simulink library "libBusSerialize"  (R2015a)
settings: Solver=ode45  StartTime=0.0  StopTime=10.0  RelTol=1e-3
undefined symbols (not defined in the file): BusSerialize, macaddr, mxpcnetworkconfig, RigInfo, SimulinkParameter_TestParamPulse, SimulinkParameter_TestParamToggle, SimulinkParameter_TunableConditions, SimulinkParameter_TunableNextTrialId, SimulinkParameter_TunableTaskControl
libraries: simulink x5, xpcethernetlib x3, xpcnetworkbufferlib x2, xpcrtudplib x1
(part 1 of 2)
settings Model: xpc_rtwmakecfg_data=_xpcetherlib__xpcether8255xlib__xpcetherGbElib__xpcnblib__xpciplib_  CovSFcnEnable=off  Creator=shenoylab  LastModifiedBy=shenoylab
settings DebuggingCC: SolverPrmCheckMsg=warning

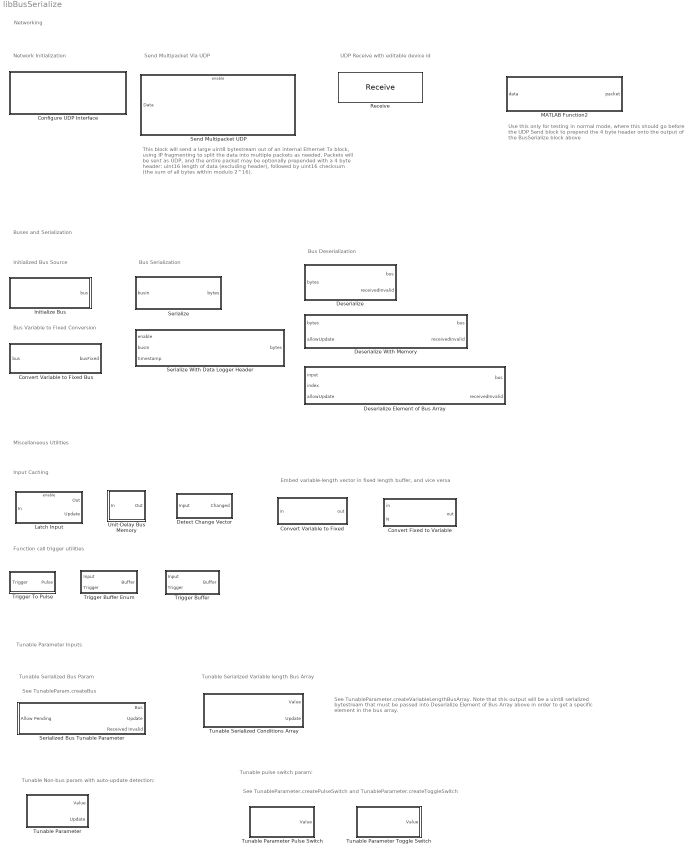
== system libBusSerialize ==
  note: See TunableParameter.createPulseSwitch and TunableParameter.createToggleSwitch
  note: See TunableParam.createBus
  note: See TunableParameter.createVariableLengthBusArray.
      | Note that this output will be a uint8 serialized bytestream that must
      | be passed into Deserialize Element of Bus Array above in order to get a
      | specific element in the bus array.
  note: Use this only for testing in normal mode,
      | where this should go before the UDP Send block
      | to prepend the 4 byte header onto the output of
      | the BusSerialize block above
  note: This block will send a large uint8 bytestream out of an
      | internal Ethernet Tx block, using IP fragmenting to split
      | the data into multiple packets as needed. Packets will be
      | sent as UDP, and the entire packet may be optionally
      | prepended with a 4 byte header: uint16 length of data
      | (excluding header), followed by uint16 checksum (the
      | sum of all bytes within modulo 2^16).
  note: Send Multipacket Via UDP
  note: Bus Serialization
  note: Bus Deserialization
  note: Bus Variable to Fixed Conversion
  note: Input Caching
  note: Function call trigger utilities
  note: Embed variable-length vector in fixed length buffer, and vice versa
  note: Initialized Bus Source
  note: Tunable Non-bus param with auto-update detection:
  note: Tunable pulse switch param:
  note: Tunable Serialized Bus Param
  note: Tunable Serialized Variable length Bus Array
  note: Network Initialization
  note: Networking
  note: Buses and Serialization
  note: Miscellaneous Utilities
  note: Tunable Parameter Inputs
  note: UDP Receive with editable device id
  Configure UDP Interface : Subsystem  InitFcn=mxpcnetworkconfig(1);  mask(xpcnwconfig){PoolSizes=[8196 512 4096 65535], ID=RigInfo.network.hapticVLAN.ethernetId, udpID=0, IpAddress=RigInfo.network.hapticVLAN.sourceIP, SubnetMask=255.255.255.0, Gateway=0.0.0.0, EthDrv=Intel 8255x, PciBus=RigInfo.network.hapticVLAN.pciBus, PciSlot=RigInfo.network.hapticVLAN.pciSlot}
      mask prompts: PoolSizes "Buffer pool sizes (256, 512, 1024, 2048):"; ID "Device ID:"; udpID "Internal UDP ID:"; IpAddress "IP Address:"; SubnetMask "Subnet Mask:"; EthDrv "Ethernet Driver:"; PciBus "PCI Bus:"; PciSlot "PCI Slot:"
      mask help: Configure network interface for real-time UDP communication
      mask init:
      | IpAddress = ipaddr(IpAddress);
      | SubnetMask = ipaddr(SubnetMask);
      | Gateway = ipaddr(Gateway);
      | set_param([gcb '/Ethernet Init '], 'ID', num2str(ID)); % update internal ID, we don't use promotion so the field can be text rather than popup
      | udpID = ID - 1;
      | [MaskDisplay] = mxpcnetworkconfig(2, ID, EthDrv, PciBus, PciSlot);
      | % set_param(gcb, 'MaskDisplay', MaskDisplay);
      mask Help: eval('xpcdoc(''RT_NETWORK_CONFIGURATION'')');
      mask TypeOptions PoolSizes: Buffer Mngmt /PoolSizes
      mask TypeOptions EthDrv: Ethernet Init /Driver
      mask Display:
      | try
      |     ipStr = BusSerialize.ipStringFromAddress(IpAddress);
      |     disp(sprintf('Real-time UDP\nConfiguration\nPCI Bus: %d Slot: %d\nDevice ID: %d\nIP Address: %s', PciBus, PciSlot, ID, ipStr));
      | catch
      |     disp('Real-time UDP\nConfiguration');
      | end
  Convert Fixed to Variable : MATLAB Function  TreatAsAtomicUnit=on  mask(Converts Variable-size to fixed-size array){bufferSize=1500}
      mask prompts: bufferSize "Buffer Size"
      mask help: Specify maximum input size.
  Convert Variable to Fixed : MATLAB Function  TreatAsAtomicUnit=on  mask(Converts Variable-size to fixed-size array){bufferSize=1000}
      mask prompts: bufferSize "Buffer Size"
      mask help: Specify maximum input size.
  Convert Variable to Fixed Bus : MATLAB Function  TreatAsAtomicUnit=on  mask(Drop Variable Length Signals From Bus){busType=Bus: TestBus, busFixedType=Bus: TestBusFixed}
      mask prompts: busType "Bus Type (Input):"; busFixedType "Bus Type (Output):"
      mask help:
      | This block takes as input a bus with some variable length signals, drops all variable length signals from the bus and outputs a bus with the specified type (second drop-down). This is accomplished by calling the appropriate model packaged code function for this bus.
      |
      | See BusSerialize.createBusBaseWorkspaceWithFixedSizeSignalsOnly and BusSerialize.writeDropVariableLengthSignalsFromBusModelPackagedCode.
      mask init:
      | BusSerialize.maskDropVariableLengthSignalsFromBusBlockUpdate(gcb)
  Deserialize : MATLAB Function  TreatAsAtomicUnit=on  mask(BusSerialize: deserialize block){busType=Bus: TestBus}
      mask prompts: busType "Bus Type"
      mask help: Select the bus type below to deserialize into.
      mask init:
      | BusSerialize.maskDeserializeBlockUpdate(gcb)
  Deserialize Element of Bus Array : MATLAB Function  TreatAsAtomicUnit=on  mask(BusSerialize: deserialize a single element of a serialized bus array){busType=Bus: TestBus, inputVariable=off}
      mask prompts: busType "Bus Type:"; inputVariable "Input Variable Length"
      mask help:
      | Given a bus array serialized with BusSerialize.serializeVariableLengthBusArray, this block deserializes a specific element of that bus array. This allows bus arrays to be deserialized even when the bus contains variable length elements (or the array is of variable length), which implies that Simulink cannot currently handle the bus array.
      |
      | Select the bus type below to deserialize into.
      mask init:
      | BusSerialize.maskDeserializeVariableLengthBusArrayBlockUpdate(gcb)
  Deserialize With Memory : MATLAB Function  TreatAsAtomicUnit=on  mask(Deserialize Bus With Internal Memory){busType=Bus: TestBus}
      mask prompts: busType "Bus Type:"
      mask help:
      | This block deserializes a uint8 bytestream into a specific bus type. When the input changes, the block will deserialize the new input, and the deserialization is successful, it will internally store the updated bus.
      |
      | If allowUpdate is high at that point, the new bus value will be output immediately and update will be driven high. If not, pendingUpdate will be driven high, and the updated bus will be held in an internal persistent variable. When allowUpdate goes high, this updated bus will be passed to the output, and update will be driven high.
      |
      | If an invalid serialized bus is received, receivedInvalid will be driven high, and the bus output will not change from its previously stored value. If the initial value sent to this block is invalid, a default initialized bus will be output with all zeros or empty bus elements.
      mask init:
      | BusSerialize.maskDeserializeMemoryBlockUpdate(gcb);
  Detect Change Vector : Subsystem
  Initialize Bus : MATLAB Function  TreatAsAtomicUnit=on  mask(Initialize Bus Block){busType=Bus: TestBus}
      mask prompts: busType "Bus Type:"
      mask help: This block simply wraps an initializeBus_BusName() function and is useful for debugging where bus inputs are required. It acts essentially like a ground source for bus types.
      mask init:
      | BusSerialize.maskInitializeBusBlockUpdate(gcb);
  Latch Input : Subsystem  TreatAsAtomicUnit=on
  MATLAB Function2 : MATLAB Function  TreatAsAtomicUnit=on
  "Receive " : xpcrtudplib/Receive   ID=1  Receive1=0.0.0.0  Receive2=Receive2  Receive3=Receive3  Receive4=Receive4  udpID=udpID  mask(rtudpreceive){maskID=1, sourceIP='0.0.0.0', Receive2=25000, Receive3=1500, Receive4=-1, udpID=0, ID=1}
      mask prompts: maskID "Device ID"; sourceIP "Source IP Address:"; Receive2 "Local (destination) port:"; Receive3 "Output port width:"; Receive4 "Sample time:"; udpID "Internal UDP ID:"; ID "Device ID:"
      mask help:
      | Receive data over UDP network.
      |
      | This block receives data on the specified local (destination) port. To receive all data sent to this port, set 'Source IP Address' to 0.0.0.0. To receive data sent to this port from a specific remote source, enter that IP address.
      mask init:
      | set(gcbh, 'ID', num2str(maskID));
      | set(gcbh, 'Receive1', sourceIP);
      mask TypeOptions Receive2: Receive2
      mask TypeOptions Receive3: Receive3
      mask TypeOptions Receive4: Receive4
      mask TypeOptions udpID: udpID
      mask TypeOptions ID: ID
      mask Display:
      | try
      |     disp(sprintf('UDP Receive\nDevice ID: %d\n%s : %d', maskID, sourceIP, Receive2));
      | catch
      |     disp('UDP Receive');
      | end
      | port_label('output', 1, 'Data');
      | port_label('output', 2, 'N');
  Send Multipacket UDP : Subsystem  mask(Send Multipacket UDP Block){transmitId=1, sourceIP=[192 168 1 1], sourcePort=20000, destIP=[192 168 1 255], destPort=25000, destMac='ff:ff:ff:ff:ff:ff', deviceID=1, prependHeader=on}
      mask prompts: transmitId "Transmit ID (must be unique):"; sourceIP "Source IP:"; sourcePort "Source Port:"; destIP "Destination IP:"; destPort "Destination Port:"; destMac "Destination MAC:"; deviceID "Ethernet Device ID:"; prependHeader "Prepend 4-byte Header (uint16 length, uint16 checksum)"
      mask help: Splits a UDP packet into multiple pieces to be reassembled at the receiver
      mask init:
      | set_param([gcb, '/Packet Iterator/Ethernet Tx '], 'ID', num2str(deviceID));
      mask Display:
      | disp(sprintf('UDP Send Multipacket\nDevice ID: %d (Transmit %d)\nFrom: %s : %d\nTo: %s : %d\nDest Mac: %s', ...
      |     deviceID, transmitId, ...
      |     BusSerialize.ipStringFromAddress(sourceIP), sourcePort, ...
      |     BusSerialize.ipStringFromAddress(destIP), destPort, destMac));
      | port_label('input', 1, 'uint8');
      | port_label('Enable','Enable')
  Serialize : MATLAB Function  TreatAsAtomicUnit=on  mask(BusSerialize: serialize block){busType=Bus: TestBus}
      mask prompts: busType "Bus Type"
      mask help: Select the bus type below to serialize.
      mask init:
      | BusSerialize.maskSerializeBlockUpdate(gcb)
  Serialize With Data Logger Header : MATLAB Function  TreatAsAtomicUnit=on  mask(BusSerialize: serialize block){busType=Bus: TestBus, groupType=Control, groupName='groupName'}
      mask prompts: busType "Bus Type"; groupType "Group Type"; groupName "Group Name"
      mask help: Select the bus type below to serialize.
      mask init:
      | BusSerialize.maskSerializeWithDataLoggerHeaderBlockUpdate(gcb)
  Serialized Bus Tunable Parameter : Subsystem  mask(BusSerialize Tunable Parameter Block){paramName='TunableTaskControl'}
      mask prompts: paramName "Parameter Name"
      mask help: This block provides the value of a tunable Simulink.Parameter into the model. Since tunable parameters with xPC target can only be doubles, the functions BusSerialize.createTunableParameter and BusSerialize.setTunableParameter automatically handle typecasting and update counter insertion, and this block handles update detection, typecasting, and reshaping back to the original form. Currently, variable size parameters are not supported.
      mask init:
      | BusSerialize.maskSerializedBusTunableParameterBlockUpdate(gcb);
      mask Display:
      | port_label('output', 1, paramName);
      | port_label('output', 2, 'Update');
      | port_label('output', 3, 'Received Invalid');
      | port_label('input', 1, 'Allow Pending');
  Trigger Buffer : Subsystem  mask(Trigger Buffer){bufferSize=100}
      mask prompts: bufferSize "Buffer Size (elements)"
      mask help: This block concatenates all inputs it receives via a function-call trigger, with the output reflecting the concatenated inputs recevied during each single tick.
  Trigger Buffer Enum : Subsystem  mask(Trigger Buffer){bufferSize=10, bufferType=Enum: TaskEvent}
      mask prompts: bufferSize "Buffer Size (elements)"; bufferType "Enum Type"
      mask help: This block concatenates all inputs it receives via a function-call trigger, with the output reflecting the concatenated inputs recevied during each single tick.
  Trigger To Pulse : Subsystem  mask(Trigger to Pulse){}
      mask help: This block converts a function-call trigger to a single-tick pulse signal which can be used as an Enable input.
  Tunable Parameter : Subsystem  mask(BusSerialize Tunable Parameter Block){paramName='TunableParam'}
      mask prompts: paramName "Parameter Name"
      mask help: This block provides the value of a tunable Simulink.Parameter into the model. Since tunable parameters with xPC target can only be doubles, the functions BusSerialize.createTunableParameter and BusSerialize.setTunableParameter automatically handle typecasting and update counter insertion, and this block handles update detection, typecasting, and reshaping back to the original form. Currently, variable size parameters are not supported.
      mask init:
      | BusSerialize.maskTunableParameterBlockUpdate(gcb);
      mask Display:
      | port_label('output', 1, paramName)
      | port_label('output', 2, 'Update');
  Tunable Parameter Pulse Switch : Subsystem  mask(BusSerialize Tunable Parameter Block){paramName='TestParamPulse'}
      mask prompts: paramName "Parameter Name"
      mask help: This block provides the value of a tunable Simulink.Parameter into the model. Since tunable parameters with xPC target can only be doubles, the functions BusSerialize.createTunableParameter and BusSerialize.setTunableParameter automatically handle typecasting and update counter insertion, and this block handles update detection, typecasting, and reshaping back to the original form. Currently, variable size parameters are not supported.
      mask init:
      | BusSerialize.maskTunableParameterPulseSwitchBlockUpdate(gcb);
      settings: OpenFcn=|
      | paramName = getBlockParamEval(gcb, 'paramName');
      | param = BusSerialize.getTunableParameterReferenceFromName(paramName);
      | param.activatePulseSwitch();
      | 
      | % turn the block green
      | setBlockParam(gcb, 'BackgroundColor', 'green');
      | 
      | % wait a bit
      | pause(0.05);
      | 
      | % and set it back to white
      | setBlockParam(gcb, 'BackgroundColor', 'lightBlue');
      mask Display: port_label('output', 1, paramName)
  Tunable Parameter Toggle Switch : Subsystem  InitFcn=|  mask(BusSerialize Tunable Parameter Block){paramName='TestParamToggle'}
      | if ~isBlockInLibrary(gcb)
      |     paramName = getBlockParamEval(gcb, 'paramName');
      |     param = BusSerialize.getTunableParameterReferenceFromName(paramName);
      |     value = param.value;
      | 
      |     if value
      |         % turn the block green
      |         setBlockParam(gcb, 'BackgroundColor', 'green');  
      |     else
      |         % keep it white
      |         setBlockParam(gcb, 'BackgroundColor', 'lightBlue');
      |     end
      | end
      mask prompts: paramName "Parameter Name"
      mask help:
      | This block provides the value of a tunable Simulink.Parameter into the model. Since tunable parameters with xPC target can only be doubles, the functions BusSerialize.createTunableParameter and BusSerialize.setTunableParameter automatically handle typecasting and update counter insertion, and this block handles update detection, typecasting, and reshaping back to the original form. Currently, variable size parameters are not supported.
      |
      | Use BusSerialize.TunableParameter.create(paramName) to create a parameter with this name.
      mask init:
      | BusSerialize.maskTunableParameterToggleSwitchBlockUpdate(gcb);
      settings: OpenFcn=|
      | if ~isBlockInLibrary(gcb)
      |     paramName = getBlockParamEval(gcb, 'paramName');
      |     param = BusSerialize.getTunableParameterReferenceFromName(paramName);
      |     value = param.toggleSwitch();
      | else
      |     value = uint8(0);
      | end
      | 
      | if value
      |     % turn the block green
      |     setBlockParam(gcb, 'BackgroundColor', 'green');
      | else
      |     % keep it white
      |     setBlockParam(gcb, 'BackgroundColor', 'lightBlue');
      | end
      mask Display: port_label('output', 1, paramName)
  Tunable Serialized Conditions Array : Subsystem  mask(BusSerialize Tunable Parameter Variable Length Bus Array Block){paramName='TunableConditions'}
      mask prompts: paramName "Parameter Name"
      mask help:
      | This block provides the value of a tunable Simulink.Parameter into the model. Since tunable parameters with xPC target can only be doubles, the functions BusSerialize.createTunableParameter and BusSerialize.setTunableParameter automatically handle typecasting and update counter insertion, and this block handles update detection, typecasting, and reshaping back to the original form. Currently, variable size parameters are not supported.
      |
      | This block specifically extracts a serialized variable length bus array, which can then be passed into the variable length bus array element extractor block.
      mask init:
      | BusSerialize.maskTunableParameterVariableLengthBusArrayBlockUpdate(gcb);
      mask Display:
      | port_label('output', 1, paramName)
      | port_label('output', 2, 'Update');
  Unit-Delay Bus Memory : Subsystem  mask(Bus Unit-Delay Memory Block){busType=Bus: RigOutputBus}
      mask prompts: busType "Bus Type:"
      mask help: This block acts exactly like a Memory block and can be used to break algebraic loops. However, unlike Memory blocks, it supports bus signals with variable length bus elements. Internally, this is done by serializing the bus, passing it through a Memory block, and then deserializing at the other end.
      mask init:
      | BusSerialize.maskBusMemoryBlockUpdate(gcb);
      mask Display:
      | text(.5, 0.2, 'Bus Memory', 'HorizontalAlignment', 'center');
      | x = [0.5 0.7 0.7 0.3 0.3 0.25 NaN 0.35 0.3];
      | y = [0.4 0.4 0.8 0.8 0.4 0.45 NaN 0.45 0.4];
      | plot(x, y);

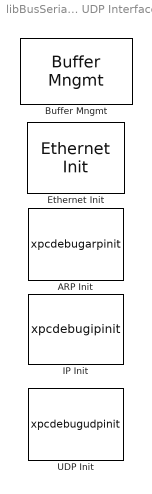
== system libBusSerialize/Configure UDP Interface ==
  "ARP Init " : S-Function  Priority=0  FunctionName=xpcdebugarpinit  Parameters=Stats, Interface, IpAddress, SubnetMask, Gateway, EthernetId, Flags, BlockId, Retry, Timeout, Expiration, StaticAddressListIp, StaticAddressListMac, DiscoveryList, MulticastList, SampleTime  mask(arpinit){Interface=udpID, IpAddress=IpAddress, SubnetMask=SubnetMask, Gateway=Gateway, EthernetId=ID, BlockId=0, SampleTime=-1, Flags=hex2dec('00000697'), Stats=off, Retry=5, Timeout=20, Expiration=20*60, StaticAddressListIp=[], StaticAddressListMac=[], DiscoveryList=[], MulticastList=[]}
      mask prompts: IpAddress "IP Address"; SubnetMask "Subnet Mask"; EthernetId "Ethernet ID"; BlockId "Block ID"; SampleTime "Sample Time"; Stats "Statistics Port"; StaticAddressListIp "[Static IP]"; StaticAddressListMac "[Static MAC]"; DiscoveryList "[Discovery IP]"; MulticastList "[Multicast IP]"
      mask help: ARP Init
      mask init:
      | xpclinklib('xpciplib');
      mask Help: web('arpdebug.htm',  '-helpbrowser');
      mask Display: disp('ARP Init');
  "Buffer Mngmt " : xpcnetworkbufferlib/Buffer Mngmt   Priority=-1  SampleTime=-1  PoolSizes=PoolSizes  ShowTune=on
  "Ethernet Init " : xpcethernetlib/Ethernet Init   Priority=-1  ID=5  Driver=Intel 8255x  Bus=PciBus  Slot=PciSlot  SampleTime=-1  AddressSource=EEPROM  MAC=macaddr('00:00:00:00:00:00')  TxSA=off  RxPromiscuous=off  Multicast={}  RxBad=off  RxShort=off  MaxMTU=1518  TxThreshold=224  TxBuffers=128  RxBuffers=64  ShowTune=off  NumRxBlks=1
  "IP Init " : S-Function  Priority=1  FunctionName=xpcdebugipinit  Parameters=Stats, Group, ArpId, IpAddress, SubnetMask, DefaultGateway, DefaultInterface, Flags, ToS, StartingId, TTL, SampleTime  mask(ipinit){Group=udpID, ArpId=[udpID], IpAddress=[IpAddress], SubnetMask=[SubnetMask], DefaultGateway=Gateway, DefaultInterface=0, SampleTime=-1, Flags=hex2dec('00000005'), ToS=hex2dec('00'), StartingId=10000, TTL=64, Stats=off}
      mask prompts: ArpId "[ARP ID]"; IpAddress "[IP Address]"; SubnetMask "[Subnet Mask]"; DefaultGateway "Default Gateway"; DefaultInterface "Default Interface"; SampleTime "Sample Time"; StartingId "Starting Id"; Stats "Statistics Port"
      mask help: IP Init
      mask init:
      | xpclinklib('xpciplib');
      mask Help: web('ipdebug.htm',  '-helpbrowser');
      mask Display: disp('IP Init');
  "UDP Init " : S-Function  Priority=2  FunctionName=xpcdebugudpinit  Parameters=Stats, Group, StartingPort, Flags, SampleTime  mask(udpinit){Group=udpID, StartingPort=10000, Flags=hex2dec('00000001'), SampleTime=-1, Stats=off}
      mask prompts: StartingPort "Starting Port"; SampleTime "Sample Time"; Stats "Statistics Port"
      mask help: UDP Init
      mask init:
      | xpclinklib('xpciplib');
      mask Help: web('udpdebug.htm',  '-helpbrowser');
      mask Display: disp('UDP Init');

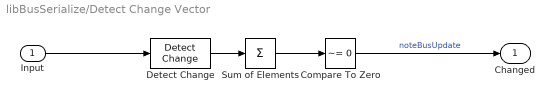
== system libBusSerialize/Detect Change Vector ==
  Input : Inport
  Compare To Zero : simulink/Logic and Bit Operations/Compare To Zero  relop=~=  OutDataTypeStr=uint8
  Detect Change : simulink/Logic and Bit Operations/Detect Change  vinit=0  InputProcessing=Inherited  OutDataTypeStr=boolean
  Sum of Elements : Sum  Inputs=+
  Changed : Outport  OutDataTypeStr=uint8
  wires:
  Sum of Elements/1 -> Compare To Zero/1
  Detect Change/1 -> Sum of Elements/1
  Compare To Zero/1 -> Changed/1  "noteBusUpdate"
  Input/1 -> Detect Change/1

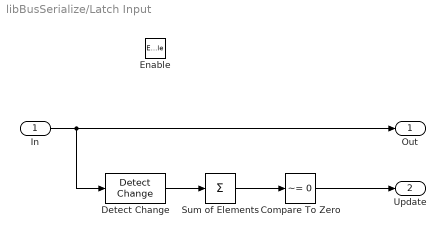
== system libBusSerialize/Latch Input ==
  In : Inport
  Enable : EnablePort
  Compare To Zero : simulink/Logic and Bit Operations/Compare To Zero  relop=~=  OutDataTypeStr=uint8  ZeroCross=off
  Detect Change : simulink/Logic and Bit Operations/Detect Change  vinit=0  InputProcessing=Inherited  OutDataTypeStr=boolean
  Sum of Elements : Sum  Inputs=+
  Out : Outport
  Update : Outport  Port=2  OutputWhenDisabled=reset  InitialOutput=0
  wires:
  In/1 -> Out/1, Detect Change/1
  Detect Change/1 -> Sum of Elements/1
  Sum of Elements/1 -> Compare To Zero/1
  Compare To Zero/1 -> Update/1

== system libBusSerialize/Send Multipacket UDP ==
  Data : Inport  OutDataTypeStr=uint8
  Enable : EnablePort  PropagateVarSize=During execution
  Compare To Zero : simulink/Logic and Bit Operations/Compare To Zero  relop=>  OutDataTypeStr=boolean
  Packet Iterator : Subsystem
  Width : Width
  wires:
  Data/1 -> Packet Iterator/1(Data), Width/1
  Width/1 -> Compare To Zero/1
  Compare To Zero/1 -> Packet Iterator/Enable

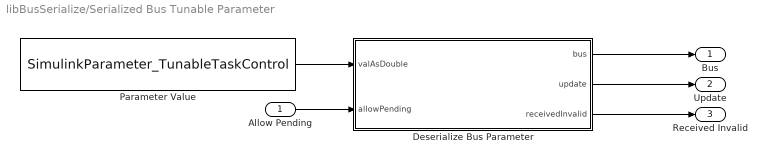
== system libBusSerialize/Serialized Bus Tunable Parameter ==
  Allow Pending : Inport
  Deserialize Bus Parameter : MATLAB Function  TreatAsAtomicUnit=on
  Parameter Value : Constant  Value=SimulinkParameter_TunableTaskControl  OutDataTypeStr=double
  Bus : Outport  PortDimensions=1
  Update : Outport  Port=2  OutDataTypeStr=uint8  PortDimensions=1
  Received Invalid : Outport  Port=3  OutDataTypeStr=uint8  PortDimensions=1
  wires:
  Deserialize Bus Parameter/2(update) -> Update/1
  Deserialize Bus Parameter/1(bus) -> Bus/1
  Deserialize Bus Parameter/3(receivedInvalid) -> Received Invalid/1
  Allow Pending/1 -> Deserialize Bus Parameter/2(allowPending)
  Parameter Value/1 -> Deserialize Bus Parameter/1(valAsDouble)

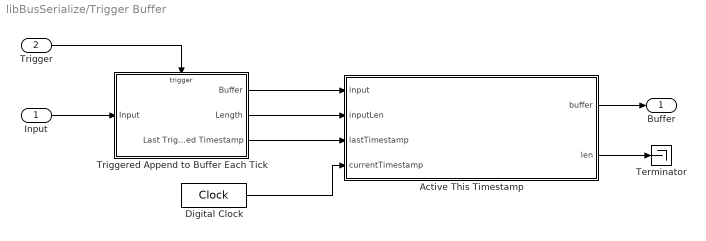
== system libBusSerialize/Trigger Buffer ==
  Input : Inport
  Trigger : Inport  Port=2
  Active This Timestamp : MATLAB Function  TreatAsAtomicUnit=on
  Digital Clock : DigitalClock  SampleTime=-1
  Terminator : Terminator
  Triggered Append to Buffer Each Tick : Subsystem
  Buffer : Outport
  wires:
  Active This Timestamp/2(len) -> Terminator/1
  Input/1 -> Triggered Append to Buffer Each Tick/1(Input)
  Triggered Append to Buffer Each Tick/3(Last Triggered Timestamp) -> Active This Timestamp/3(lastTimestamp)
  Triggered Append to Buffer Each Tick/2(Length) -> Active This Timestamp/2(inputLen)
  Triggered Append to Buffer Each Tick/1(Buffer) -> Active This Timestamp/1(input)
  Active This Timestamp/1(buffer) -> Buffer/1
  Digital Clock/1 -> Active This Timestamp/4(currentTimestamp)
  Trigger/1 -> Triggered Append to Buffer Each Tick/Trigger

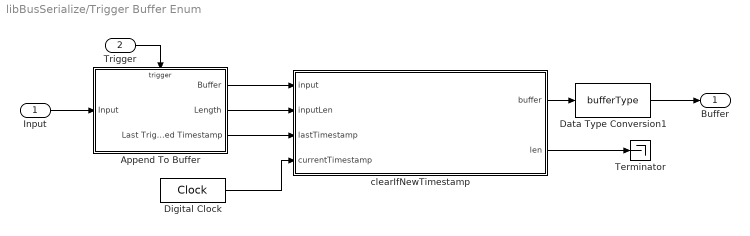
== system libBusSerialize/Trigger Buffer Enum ==
  Input : Inport  OutDataTypeStr=bufferType
  Trigger : Inport  Port=2
  Append To Buffer : Subsystem
  Data Type Conversion1 : DataTypeConversion  OutDataTypeStr=bufferType
  Digital Clock : DigitalClock  SampleTime=-1
  Terminator : Terminator
  clearIfNewTimestamp : MATLAB Function  TreatAsAtomicUnit=on
  Buffer : Outport  OutDataTypeStr=bufferType
  wires:
  Input/1 -> Append To Buffer/1(Input)
  clearIfNewTimestamp/1(buffer) -> Data Type Conversion1/1
  Data Type Conversion1/1 -> Buffer/1
  Trigger/1 -> Append To Buffer/Trigger
  Digital Clock/1 -> clearIfNewTimestamp/4(currentTimestamp)
  Append To Buffer/1(Buffer) -> clearIfNewTimestamp/1(input)
  Append To Buffer/2(Length) -> clearIfNewTimestamp/2(inputLen)
  Append To Buffer/3(Last Triggered Timestamp) -> clearIfNewTimestamp/3(lastTimestamp)
  clearIfNewTimestamp/2(len) -> Terminator/1

== system libBusSerialize/Trigger To Pulse ==
  Trigger : Inport
  Active This Timestamp : MATLAB Function  TreatAsAtomicUnit=on
  Capture timestamp : Subsystem
  Digital Clock : DigitalClock  SampleTime=-1
  Pulse : Outport
  wires:
  Active This Timestamp/1(active) -> Pulse/1
  Digital Clock/1 -> Active This Timestamp/2(currentTimestamp)
  Capture timestamp/1(Last Triggered Timestamp) -> Active This Timestamp/1(lastTimestamp)
  Trigger/1 -> Capture timestamp/Trigger

== system libBusSerialize/Tunable Parameter ==
  Deserialize Parameter : MATLAB Function  TreatAsAtomicUnit=on
  Parameter Value : Constant  Value=SimulinkParameter_TunableNextTrialId  OutDataTypeStr=double
  Value : Outport
  Update : Outport  Port=2
  wires:
  Deserialize Parameter/1(value) -> Value/1
  Deserialize Parameter/2(update) -> Update/1
  Parameter Value/1 -> Deserialize Parameter/1(valAsDouble)

== system libBusSerialize/Tunable Parameter Pulse Switch ==
  Deserialize Parameter : MATLAB Function  TreatAsAtomicUnit=on
  Parameter Value : Constant  Value=SimulinkParameter_TestParamPulse  OutDataTypeStr=double
  Terminator : Terminator
  Value : Outport  OutDataTypeStr=uint8  PortDimensions=1
  wires:
  Deserialize Parameter/1(value) -> Value/1
  Deserialize Parameter/2(update) -> Terminator/1
  Parameter Value/1 -> Deserialize Parameter/1(valAsDouble)

== system libBusSerialize/Tunable Parameter Toggle Switch ==
  Deserialize Parameter : MATLAB Function  TreatAsAtomicUnit=on
  Parameter Value : Constant  Value=SimulinkParameter_TestParamToggle  OutDataTypeStr=double
  Terminator : Terminator
  Value : Outport  OutDataTypeStr=uint8  PortDimensions=1
  wires:
  Deserialize Parameter/1(value) -> Value/1
  Deserialize Parameter/2(update) -> Terminator/1
  Parameter Value/1 -> Deserialize Parameter/1(valAsDouble)

== system libBusSerialize/Tunable Serialized Conditions Array ==
  Deserialize Parameter : MATLAB Function  TreatAsAtomicUnit=on
  Parameter Value : Constant  Value=SimulinkParameter_TunableConditions  OutDataTypeStr=double
  Value : Outport
  Update : Outport  Port=2
  wires:
  Parameter Value/1 -> Deserialize Parameter/1(valAsDouble)
  Deserialize Parameter/2(update) -> Update/1
  Deserialize Parameter/1(value) -> Value/1

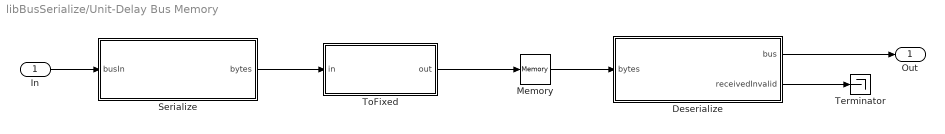
== system libBusSerialize/Unit-Delay Bus Memory ==
  In : Inport  OutDataTypeStr=Bus: RigOutputBus  PortDimensions=1
  Deserialize : MATLAB Function  TreatAsAtomicUnit=on  mask(BusSerialize: deserialize block){busType=Bus: RigOutputBus}
      mask prompts: busType "Bus Type"
      mask help: Select the bus type below to deserialize into.
      mask init:
      | BusSerialize.maskDeserializeBlockUpdate(gcb)
  Memory : Memory
  Serialize : MATLAB Function  TreatAsAtomicUnit=on  mask(BusSerialize: serialize block){busType=Bus: RigOutputBus}
      mask prompts: busType "Bus Type"
      mask help: Select the bus type below to serialize.
      mask init:
      | BusSerialize.maskSerializeBlockUpdate(gcb)
  Terminator : Terminator
  ToFixed : MATLAB Function  TreatAsAtomicUnit=on  mask(Converts Variable-size to fixed-size array){bufferSize=173164}
      mask prompts: bufferSize "Buffer Size"
      mask help: Specify maximum input size.
  Out : Outport  OutDataTypeStr=Bus: RigOutputBus
  wires:
  ToFixed/1(out) -> Memory/1
  Serialize/1(bytes) -> ToFixed/1(in)
  Memory/1 -> Deserialize/1(bytes)
  In/1 -> Serialize/1(busIn)
  Deserialize/2(receivedInvalid) -> Terminator/1
  Deserialize/1(bus) -> Out/1

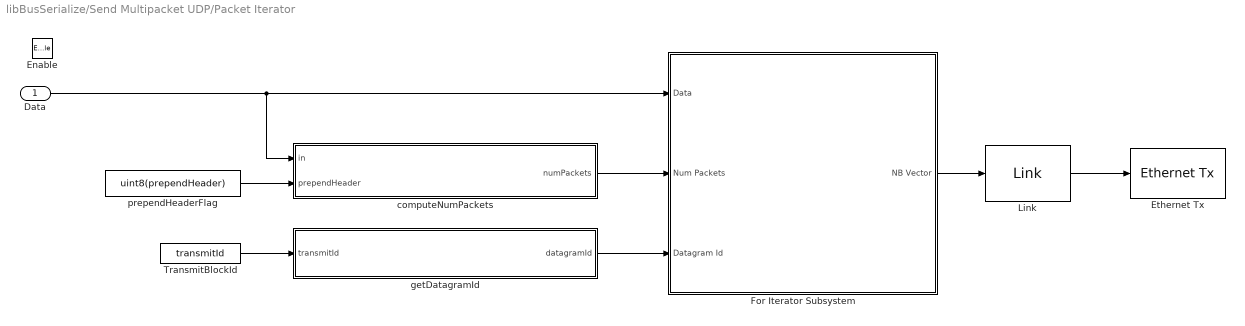
== system libBusSerialize/Send Multipacket UDP/Packet Iterator ==
  Data : Inport
  Enable : EnablePort  PropagateVarSize=During execution
  "Ethernet Tx " : xpcethernetlib/Ethernet Tx   ID=1  SampleTime=-1
  For Iterator Subsystem : Subsystem  TreatAsAtomicUnit=on
  "Link " : xpcnetworkbufferlib/Link 
  TransmitBlockId : Constant  Value=transmitId  OutDataTypeStr=uint8
  computeNumPackets : MATLAB Function  TreatAsAtomicUnit=on
  getDatagramId : MATLAB Function  TreatAsAtomicUnit=on
  prependHeaderFlag : Constant  Value=uint8(prependHeader)  OutDataTypeStr=uint8
  wires:
  computeNumPackets/1(numPackets) -> For Iterator Subsystem/2(Num Packets)
  prependHeaderFlag/1 -> computeNumPackets/2(prependHeader)
  getDatagramId/1(datagramId) -> For Iterator Subsystem/3(Datagram Id)
  For Iterator Subsystem/1(NB Vector) -> "Link "/1
  TransmitBlockId/1 -> getDatagramId/1(transmitId)
  "Link "/1 -> "Ethernet Tx "/1
  Data/1 -> For Iterator Subsystem/1(Data), computeNumPackets/1(in)

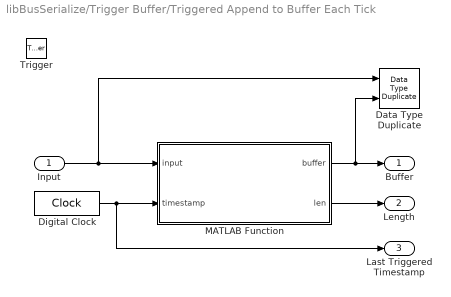
== system libBusSerialize/Trigger Buffer/Triggered Append to Buffer Each Tick ==
  Input : Inport
  Trigger : TriggerPort  TriggerType=function-call  StatesWhenEnabling=reset  PortDimensions=1
  Data Type Duplicate : DataTypeDuplicate
  Digital Clock : DigitalClock  SampleTime=-1
  MATLAB Function : MATLAB Function  TreatAsAtomicUnit=on
  Buffer : Outport
  Length : Outport  Port=2
  Last Triggered Timestamp : Outport  Port=3
  wires:
  Digital Clock/1 -> MATLAB Function/2(timestamp), Last Triggered Timestamp/1
  Input/1 -> MATLAB Function/1(input), Data Type Duplicate/1
  MATLAB Function/1(buffer) -> Buffer/1, Data Type Duplicate/2
  MATLAB Function/2(len) -> Length/1

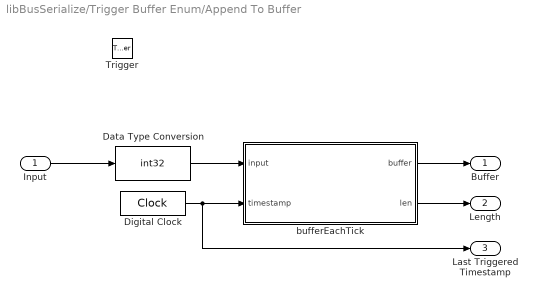
== system libBusSerialize/Trigger Buffer Enum/Append To Buffer ==
  Input : Inport  OutDataTypeStr=bufferType
  Trigger : TriggerPort  TriggerType=function-call  StatesWhenEnabling=reset  PortDimensions=1
  Data Type Conversion : DataTypeConversion  OutDataTypeStr=int32
  Digital Clock : DigitalClock  SampleTime=-1
  bufferEachTick : MATLAB Function  TreatAsAtomicUnit=on
  Buffer : Outport  OutDataTypeStr=int32
  Length : Outport  Port=2
  Last Triggered Timestamp : Outport  Port=3
  wires:
  bufferEachTick/2(len) -> Length/1
  bufferEachTick/1(buffer) -> Buffer/1
  Digital Clock/1 -> Last Triggered Timestamp/1, bufferEachTick/2(timestamp)
  Data Type Conversion/1 -> bufferEachTick/1(input)
  Input/1 -> Data Type Conversion/1

== system libBusSerialize/Trigger To Pulse/Capture timestamp ==
  Trigger : TriggerPort  TriggerType=function-call  StatesWhenEnabling=reset  PortDimensions=1
  Digital Clock : DigitalClock  SampleTime=-1
  Last Triggered Timestamp : Outport  OutputWhenDisabled=reset  InitialOutput=-1
  wires:
  Digital Clock/1 -> Last Triggered Timestamp/1

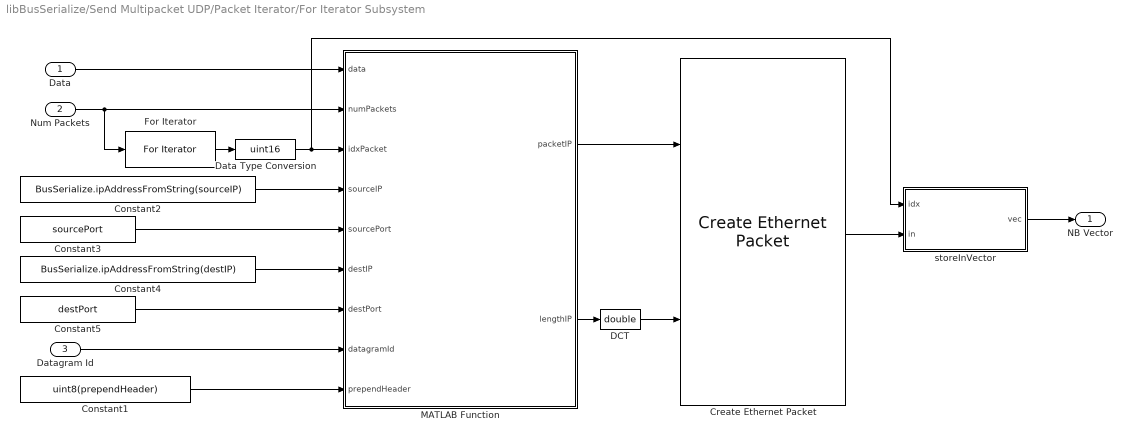
== system libBusSerialize/Send Multipacket UDP/Packet Iterator/For Iterator Subsystem ==
  Data : Inport  OutDataTypeStr=uint8
  Num Packets : Inport  Port=2  OutDataTypeStr=uint16  PortDimensions=1
  Datagram Id : Inport  Port=3  OutDataTypeStr=uint8  PortDimensions=2
  Constant1 : Constant  Value=uint8(prependHeader)  OutDataTypeStr=uint8
  Constant2 : Constant  Value=BusSerialize.ipAddressFromString(sourceIP)  OutDataTypeStr=uint8
  Constant3 : Constant  Value=sourcePort  OutDataTypeStr=uint16
  Constant4 : Constant  Value=BusSerialize.ipAddressFromString(destIP)  OutDataTypeStr=uint8
  Constant5 : Constant  Value=destPort  OutDataTypeStr=uint16
  "Create Ethernet Packet " : xpcethernetlib/Create Ethernet Packet   DstMac=macaddr(destMac)  EtherType=hex2dec('0800')
  DCT : DataTypeConversion  OutDataTypeStr=double
  Data Type Conversion : DataTypeConversion  OutDataTypeStr=uint16
  For Iterator : ForIterator  IterationSource=external  IterationVariableDataType=int16
  MATLAB Function : MATLAB Function  TreatAsAtomicUnit=on
  storeInVector : MATLAB Function  TreatAsAtomicUnit=on
  NB Vector : Outport
  wires:
  storeInVector/1(vec) -> NB Vector/1
  "Create Ethernet Packet "/1 -> storeInVector/2(in)
  Datagram Id/1 -> MATLAB Function/8(datagramId)
  Constant2/1 -> MATLAB Function/4(sourceIP)
  Constant3/1 -> MATLAB Function/5(sourcePort)
  Constant5/1 -> MATLAB Function/7(destPort)
  DCT/1 -> "Create Ethernet Packet "/2
  MATLAB Function/1(packetIP) -> "Create Ethernet Packet "/1
  MATLAB Function/2(lengthIP) -> DCT/1
  Constant1/1 -> MATLAB Function/9(prependHeader)
  Constant4/1 -> MATLAB Function/6(destIP)
  Data/1 -> MATLAB Function/1(data)
  Data Type Conversion/1 -> storeInVector/1(idx), MATLAB Function/3(idxPacket)
  Num Packets/1 -> For Iterator/1, MATLAB Function/2(numPackets)
  For Iterator/1 -> Data Type Conversion/1

== matlab function libBusSerialize/Tunable Parameter/Deserialize Parameter ==
  data: valAsDouble input double; value output uint32 size=[1 1]; update output uint8 size=1
function [value, update] = deserializeParameter(valAsDouble)
%#codegen

valAsBytes = typecast(valAsDouble, 'uint8');

% check for whether counter has been incremented
thisCounter = valAsBytes(1);
persistent pLastCounter;
if isempty(pLastCounter)
    pLastCounter = thisCounter;
end
if pLastCounter ~= thisCounter
    update = uint8(1);
    pLastCounter = thisCounter;
else
    update = uint8(0);
end

% typecast and reshape the value
value = reshape(typecast(valAsBytes(double(2):double(5)), 'uint32'), [1 1]);

== matlab function libBusSerialize/MATLAB Function2 ==
  data: data input uint8; packet output uint8 size=65000
function packet = prependLengthChecksumHeader(data)
%#codegen

% 8 byte header on first packet containing '#udp', 2 byte length, 2 byte checksum

coder.varsize('packet', 65000);

% include custom 8 byte custom header with length and checksum
headerPre = zeros(4, 1, 'uint8');
headerPre(1:2) = typecast(uint16(numel(data)), 'uint8');
checksum = uint16(mod(sum(uint32(data)), uint32(65536)));
headerPre(3:4) = typecast(checksum, 'uint8');
packet = [headerPre; data];

== matlab function libBusSerialize/Send Multipacket UDP/Packet Iterator/For Iterator Subsystem/MATLAB Function ==
  data: data input uint8; numPackets input uint16 size=1; idxPacket input uint16 size=1; packetIP output uint8; lengthIP output uint16 size=1; sourceIP input uint8 size=4; sourcePort input uint16 size=1; destIP input uint8 size=4; destPort input uint16; datagramId input; prependHeader input
function [packetIP, lengthIP] = buildSubPacket(data, numPackets, idxPacket, sourceIP, sourcePort, destIP, destPort, datagramId, prependHeader)
%#codegen
% Creates a single UDP/IP packet that transmits one fragment of a possibly
% multi-fragment set of IP packets carrying the payload in data. idxPacket
% is the index of the fragment to send (1-indexed), out of num packets
% total fragments.
%
% Inputs:  
%   data : uint8 Nx1 or 1xN packet data vectors
%   numPackets, idxPacket : uint16 scalars
%   sourceIP, destIP : 1x4 uint8 of the IP (in address order)
%   sourcePort, destPort : uint16 port numbers
%   datagramId : uint16 scalar, unique id for this set of packets, for this timestep
%    that is used by the receiving IP stack to reassemble fragments
%   prependHeader : uint8 flag determining whether to prepend a 4 byte
%     header containing a 2 byte data length (excluding the header) and a 2
%     byte checksum (sum of bytes modulo 65536) of the data (excluding the 
%     header)
%
% Outputs:
%   packetIP : uint8 1500x1 IP packet to be passed into Create Ethernet
%     Packet block
%   lengthIP : uint16 scalar indicating the total length of packetIP
%     utilized, guaranteed to be even
% 
% Dan O'Shea, Paul Nuyujukian, Vikash Gilja
%

%% Initialize and return early if empty
packetIP = zeros(1500, 1, 'uint8');
lengthIP = uint16(0);

dataLength = numel(data);
if dataLength == 0
    return;
end

%% Build UDP subpacket

packetUDP = zeros(1480, 1, 'uint8');

% 1472 bytes per fragment
bytesPerFragment = uint16(1480);
headerUdpLength = uint16(8);
if prependHeader
    % 6 byte header on first packet containing '#u', 2 byte length, 2 byte checksum
    headerPreLength = uint16(4);
else
    headerPreLength = uint16(0);
end

headerLength = headerPreLength + headerUdpLength;

fragment = zeros(bytesPerFragment, 1, 'uint8');

% slice out the portion of data that goes in this packet
if idxPacket == 1
    byteStart = uint16(1);
    bytesThisFragment = bytesPerFragment - headerLength;
else
    % the first packet only graps 1480-8 bytes
    byteStart = uint16((idxPacket-uint16(1)) * bytesPerFragment - headerLength + uint16(1));
    bytesThisFragment = bytesPerFragment;
end

if byteStart > numel(data)
    % shouldn't happen, means idxPacket was too high for data
    return;
end
byteEnd = byteStart + bytesThisFragment - uint16(1);
% truncate fragment to data length
if byteEnd > numel(data)
    byteEnd = uint16(numel(data));
end
bytesThisFragment = byteEnd - byteStart + 1;

fragment(1:bytesThisFragment) = data(byteStart : byteEnd);

if idxPacket == 1
    if prependHeader
        headerPre = zeros(headerPreLength, 1, 'uint8');
        % 2 byte length
        headerPre(1:2) = typecast(uint16(numel(data)), 'uint8');
        % 2 byte modular checksum
        checksum = uint16(mod(uint32(sum(data)), uint32(65536)));
        headerPre(3:4) = typecast(checksum, 'uint8');
    else
        headerPre = zeros(0, 1, 'uint8');
    end
        
    % include 8 byte udp header
    headerUdp = zeros(8, 1, 'uint8');
    FFFF = uint16(hex2dec('FFFF'));
    protocol = uint8(hex2dec('11'));
    length_BE = (typecast(uint16(numel(data)) + headerLength, 'uint8')); % flip to big endian
    length_BE = length_BE(end:-1:1);
    sourcePort_BE = (typecast(sourcePort, 'uint8'));
    sourcePort_BE = sourcePort_BE(end:-1:1);
    destPort_BE   = (typecast(destPort,   'uint8'));
    destPort_BE = destPort_BE(end:-1:1);
    headerUdp(1:8) = [sourcePort_BE destPort_BE length_BE uint8([0 0])];
    pseudoHeader = [sourceIP' destIP' uint8(0) protocol length_BE];
    
    if prependHeader
        % include 4 byte header in checksum
        if floor(double(numel(data)) / 2.0) ~= double(numel(data)) / 2.0
            % data is odd length, pad with zero byte
            checksumUdp = FFFF - uint16(mod( uint32(sum( typecast([pseudoHeader headerUdp' headerPre' data(:)' uint8(0)], 'uint16') )), uint32(FFFF) ));
        else
            checksumUdp = FFFF - uint16(mod( uint32(sum( typecast([pseudoHeader headerUdp' headerPre' data(:)'], 'uint16') )), uint32(FFFF) ));
        end
    else
        if floor(double(numel(data)) / 2.0) ~= double(numel(data)) / 2.0
            % data is odd length, pad with zero byte
            checksumUdp = FFFF - uint16(mod( uint32(sum( typecast([pseudoHeader headerUdp' data(:)' uint8(0)], 'uint16') )), uint32(FFFF) ));
        else
            checksumUdp = FFFF - uint16(mod( uint32(sum( typecast([pseudoHeader headerUdp' data(:)'], 'uint16') )), uint32(FFFF) ));
        end
    end
    headerUdp(7:8) = typecast(checksumUdp, 'uint8');

    % include custom 4 byte custom header with length and checksum
    if prependHeader
        lengthUDP = uint16(numel(headerUdp) + numel(headerPre) + bytesThisFragment);
        packetUDP(1:lengthUDP) = [headerUdp; headerPre; fragment(1:bytesThisFragment)];
    else
        % no header
        lengthUDP = uint16(numel(headerUdp) + bytesThisFragment);
        packetUDP(1:lengthUDP) = [headerUdp; fragment(1:bytesThisFragment)];
    end
else
    lengthUDP = uint16(bytesThisFragment);
    packetUDP(1:lengthUDP) = fragment(1:bytesThisFragment);
end

%% Build the fragment information that goes into IP header

% first 3 bits are 0, 1=DF, 2=More Fragments
% next 15 bits are length of fragment in bytes / 8
if idxPacket == 1
    fragmentWord = uint16(0);
else
    fragmentWord = (byteStart - uint16(1) + headerLength) / uint16(8);
end
if idxPacket < numPackets
    % set the more fragments bit
    fragmentWord = bitset(fragmentWord, 14);
end

% swap to big endian
fragmentBytes = typecast(fragmentWord, 'uint8')';
fragmentBytes = fragmentBytes([2;1]);

%% Build IP packet for this fragment

% make udp content length even
if floor(double(lengthUDP) / 2) ~= (double(lengthUDP) / 2)
    lengthUDP = lengthUDP + uint16(1);
end

% build IP header
lengthIP = lengthUDP + uint16(20);
version_IHL = uint8(69); % IPv4 and IP header length of 5
ToS = uint8(0); % no QOS on network

length_BE = (typecast(lengthIP, 'uint8')); % change to big endian
length_BE = length_BE(end:-1:1);

%ff = [ uint8(bin2dec('01000000')) 0 ]; % don't fragment packets
ff = fragmentBytes';
TTL = uint8(10); % ttl to 10 seconds/hops
protocol = uint8(hex2dec('11')); % UDP Protocol
headerIP = [ version_IHL ToS length_BE datagramId' ff TTL protocol 0 0 sourceIP' destIP'];

FFFF = uint16(hex2dec('FFFF'));
checksum = FFFF - uint16(mod( uint32(sum( typecast(headerIP, 'uint16') )), uint32(FFFF) ));
headerIP(11:12) = typecast(checksum, 'uint8');

% assemble the final packet
packetIP(1:lengthIP) = [ headerIP'; packetUDP(1:lengthUDP) ];

== matlab function libBusSerialize/Send Multipacket UDP/Packet Iterator/computeNumPackets ==
  data: in input; numPackets output uint16 size=1; prependHeader input
function numPackets = computeNumPackets(in, prependHeader)
%#codegen

if numel(in) == 0
    numPackets = uint16(0);
else
    % Assuming 1500 MTU, 1480 bytes per IP packet
    % 8 bytes in udp header + 4 bytes in custom header if used, but only on the
    % first fragment sent
    if prependHeader
        headerLength = 8 + 4;
    else
        headerLength = 8;
    end
    numPackets = uint16(ceil((double(numel(in))+headerLength) / 1480));
end

== matlab function libBusSerialize/Deserialize ==
  data: bytes input; bus output Bus: TestBus size=1; receivedInvalid output uint8 size=1
function [bus, receivedInvalid] = deserializeWithMemory(bytes)

%#codegen



    % cache input so we only deserialize when input changes

    persistent pBytes;

    if isempty(pBytes)

        pBytes = bytes;

        inChanged = uint8(1);

    elseif ~isequal(pBytes, bytes)

        pBytes = bytes;

        inChanged = uint8(1);

    else

        inChanged = uint8(0);

    end

    

    persistent pInvalid;

    if isempty(pInvalid)

        pInvalid = uint8(0);

    end



    % external cached output

    persistent pBusOut;

    if isempty(pBusOut)

        pBusOut = initializeBus_TestBus();

    end



    % handle deserialization if changed

    if inChanged

        [tempBus, valid] = deserializeBus_TestBus(bytes);

        if valid

            pBusOut = tempBus;

            pInvalid = uint8(0);

        else

            pInvalid = uint8(1);

        end

    end

         

    bus = pBusOut;

    receivedInvalid = pInvalid;

end

== matlab function libBusSerialize/Serialize ==
  data: busIn input Bus: TestBus size=1; bytes output uint8 size=0
function bytes = serialize(busIn)

%#codegen 



    bytes = serializeBus_TestBus(busIn);



end

== matlab function libBusSerialize/Serialize With Data Logger Header ==
  data: enable input uint8 size=1; busIn input Bus: TestBus size=1; bytes output uint8 size=23; timestamp input uint32 size=1
function bytes = dataLoggerSerialize(enable, busIn, timestamp)
%#codegen
    if enable
        bytes = serializeBusWithDataLoggerHeader_TestBus(busIn, uint8(BusSerialize.GroupTypes.Control), uint8('groupName'), timestamp);
    else
        bytes = zeros(0, 1, 'uint8');
    end
end

== matlab function libBusSerialize/Send Multipacket UDP/Packet Iterator/getDatagramId ==
  data: transmitId input uint8 size=1; datagramId output uint8 size=2
function datagramId = getDatagramId(transmitId)
%#codegen

% generates a unique id for this block, for this packet

persistent pId
if isempty(pId)
    pId = uint8(1);
elseif pId == uint8(255)
    pId = uint8(1);
else
    pId = pId + uint8(1);
end

datagramId = [transmitId; pId];

== matlab function libBusSerialize/Send Multipacket UDP/Packet Iterator/For Iterator Subsystem/storeInVector ==
  data: idx input; vec output; in input
function vec = storeInVector(idx, in)
%#codegen

nPacketsMax = 15;

persistent pVec;
if isempty(pVec) || idx == 1
    pVec = repmat(in*0, nPacketsMax, 1);
end
if idx >= 1 && idx <= nPacketsMax
    pVec(idx) = in;
end

vec = pVec;

== matlab function libBusSerialize/Deserialize With Memory ==
  data: bytes input; bus output Bus: TestBus size=1; allowUpdate input uint8 size=1; receivedInvalid output uint8 size=1
function [bus, receivedInvalid] = deserializeWithMemory(bytes, allowUpdate)
%#codegen

    % external cached output
    persistent pBusOut;
    if isempty(pBusOut)
        pBusOut = initializeBus_TestBus();
    end

    receivedInvalid = uint8(1);

    receivedInvalid = uint8(0);
    if allowUpdate
        [bus, valid] = deserializeBus_TestBus(bytes);
        if valid
            % update internal cache
            pBusOut = bus;
        else
            % don't update internal cache, output internal cache
            bus = pBusOut;
            receivedInvalid = uint8(1);
        end
    else
        bus = pBusOut;
    end
end

== matlab function libBusSerialize/Deserialize Element of Bus Array ==
  data: input input; bus output Bus: TestBus size=1; index input uint16 size=1; allowUpdate input uint8 size=1; receivedInvalid output uint8 size=1
function [bus, receivedInvalid] = deserializeBusArrayElement(input, index, allowUpdate)
%#codegen

    in = typecast(input, 'uint8');
    receivedInvalid = uint8(0);
    valid = uint8(0);

    % cached output for allowUpdate
    persistent pBus;
    
    % cache outputs so that we only update when allowUpdate is high
    if isempty(pBus)
        pBus = initializeBus_TestBus();        
    end
    
    % deserialize a new output if we're allowing updates
    if allowUpdate

        % length is first uint16
        N = typecast(in(1:2), 'uint16');
        if index <= N
            % followed by N uint32s indicating where each element starts
            idxOffset = uint32((index-1)*4 + 3); % first offset at byte 3, second at byte 7
            if idxOffset <= length(in) % too short to hold that many?
                % get the offset where the requested bus element starts
                offset = typecast(in(idxOffset : (idxOffset + 3)), 'uint32');
                if offset <= length(in) % offset invalid?

                    % and deserialize the bus from that offset
                    [bus, valid] = deserializeBus_TestBus(in, offset);
                    if valid
                        % cache as new output
                        pBus = bus;
                    end
                end
            end
        end

        if ~valid
            % don't update cache, restore old output
            receivedInvalid = uint8(1);
        end
    end

    bus = pBus;
end

== matlab function libBusSerialize/Convert Variable to Fixed Bus ==
  data: bus input Bus: TestBus size=1; busFixed output Bus: TestBusFixed size=1
function busFixed = convertToTestBusFixed(bus)

%#codegen



    busFixed = dropVariableLengthSignalsFromBus_TestBus(bus);



end

== matlab function libBusSerialize/Trigger Buffer Enum/Append To Buffer/bufferEachTick ==
  data: input input int32; buffer output int32 size=bufferSize; timestamp input; len output uint32 size=1; bufferSize parameter size=1
function [buffer, len] = bufferEachTick(input, timestamp, bufferSize)
%#codegen

persistent pBuffer;
persistent pLastTimestamp;

coder.varsize('pBuffer', bufferSize, true);

clear = uint8(0);

% initialize persistents
if isempty(pBuffer) || isempty(pLastTimestamp)
    pBuffer = zeros(0, 1, class(input)); %#ok<ZEROLIKE>
    pLastTimestamp = timestamp;
end

% determine if this is a new tick and reset the output if it is
if pLastTimestamp ~= timestamp
    pLastTimestamp = timestamp;
    clear = uint8(1);
end

if clear
    pBuffer = input(:);
elseif numel(pBuffer) == 0
    pBuffer = input(:);
elseif numel(pBuffer) + numel(input) < bufferSize
    pBuffer = [pBuffer; input(:)];
end

buffer = pBuffer;
len = uint32(numel(buffer));

== matlab function libBusSerialize/Trigger Buffer Enum/clearIfNewTimestamp ==
  data: input input int32 size=bufferSize; inputLen input uint32 size=1; buffer output int32 size=bufferSize; lastTimestamp input; currentTimestamp input size=1; len output uint32 size=1
function [buffer, len]   = clearIfNewTimestamp(input, inputLen, lastTimestamp, currentTimestamp)
%#codegen

if lastTimestamp == currentTimestamp
    buffer = input;
    len = inputLen;
else
    buffer = zeros(0, 1, class(input));
    len = zeros(1, 1, class(inputLen)); %#ok<ZEROLIKE>
end

== matlab function libBusSerialize/Trigger To Pulse/Active This Timestamp ==
  data: active output uint8 size=1; lastTimestamp input; currentTimestamp input size=1
function active  = clearIfNewTimestamp(lastTimestamp, currentTimestamp)
%#codegen

if lastTimestamp == currentTimestamp
    active = uint8(1);
else
    active = uint8(0);
end
